simulink model "vibration_test"  (R2015b)
settings: Solver=FixedStepAuto  StartTime=0.0  StopTime=20  FixedStep=0.0001  RelTol=1e-3
settings Model: Creator=YogurtSuee  LastModifiedBy=YogurtSuee

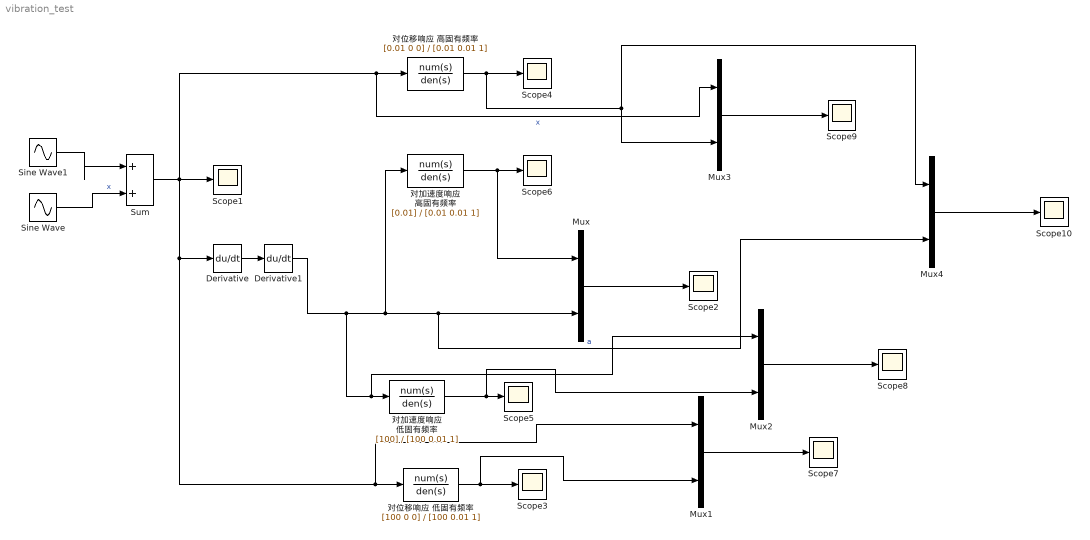
== system vibration_test ==
  Derivative : Derivative
  Derivative1 : Derivative  CoefficientInTFapproximation=Inf
  Mux{,1..4} (5 alike) : Mux  Inputs=2
  Scope{1..10} (10 alike) : Scope
  Sine Wave : Sin  SampleTime=0
  Sine Wave1 : Sin  Amplitude=0.2  Frequency=20  SampleTime=0
  Sum : Sum  Inputs=|++
  对位移响应 低固有频率 : TransferFcn  Numerator=[100 0 0]  Denominator=[100 0.01 1]
  对位移响应 高固有频率 : TransferFcn  Numerator=[0.01 0 0]  Denominator=[0.01 0.01 1]
  对加速度响应 低固有频率 : TransferFcn  Numerator=[100]  Denominator=[100 0.01 1]
  对加速度响应 高固有频率 : TransferFcn  Numerator=[0.01]  Denominator=[0.01 0.01 1]
  wires:
  Sine Wave/1 -> Sum/2  "x"
  Derivative1/1 -> Mux2/1, 对加速度响应 低固有频率/1, 对加速度响应 高固有频率/1, Mux4/2, Mux/2  "a"
  Sine Wave1/1 -> Sum/1
  Sum/1 -> Mux3/1, 对位移响应 高固有频率/1, Scope1/1, Mux1/1, 对位移响应 低固有频率/1, Derivative/1  "x"
  对位移响应 低固有频率/1 -> Mux1/2, Scope3/1
  对位移响应 高固有频率/1 -> Mux4/1, Mux3/2, Scope4/1
  对加速度响应 高固有频率/1 -> Mux/1, Scope6/1
  Derivative/1 -> Derivative1/1
  Mux/1 -> Scope2/1
  Mux1/1 -> Scope7/1
  Mux2/1 -> Scope8/1
  对加速度响应 低固有频率/1 -> Mux2/2, Scope5/1
  Mux3/1 -> Scope9/1
  Mux4/1 -> Scope10/1
